simulink model "laser_cnc_camera_pid"  (R2024a)
settings: Solver=ode23t  StartTime=0.0  StopTime=0.6  RelTol=1e-3
libraries: slpidlib x1
settings Model: Creator=Sir Kiru  LastModifiedBy=Sir Kiru

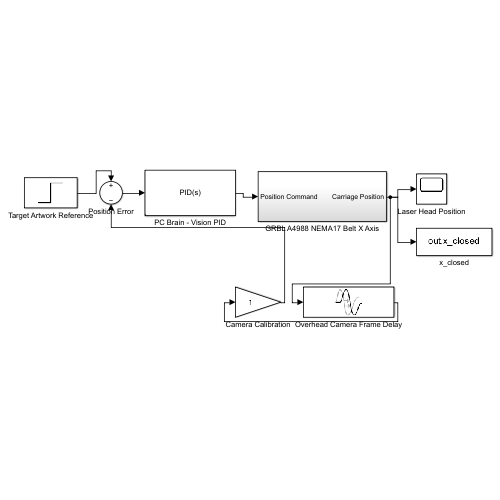
[thumbnail: Simulink's stored preview of the top-level diagram]
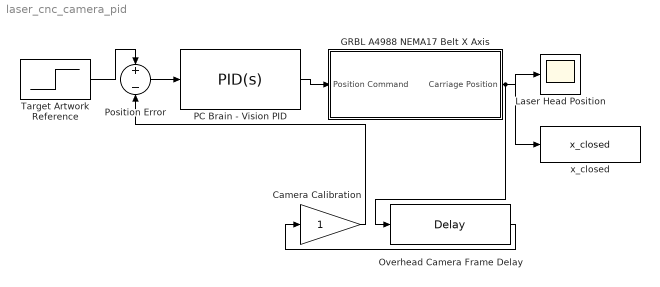
== system laser_cnc_camera_pid ==
  Camera Calibration : Gain
  GRBL A4988 NEMA17 Belt X Axis : Subsystem
  Laser Head Position : Scope
  Overhead Camera Frame Delay : TransportDelay  DelayTime=0.02
  PC Brain - Vision PID : slpidlib/PID Controller  Controller=PID  Form=Parallel  TimeDomain=Continuous-time  UseExternalTs=off  SampleTime=-1  IntegratorMethod=Forward Euler  FilterMethod=Forward Euler  ControllerParametersSource=internal  P=9  I=6  UseKiTs=off  D=0.16  UseExternalDerivativeSource=off  N=100  UseFilter=on  TunerSelectOption=Transfer Function Based (PID Tuner App)  InitialConditionSource=internal  InitialConditionForIntegrator=0  InitialConditionForFilter=0  DifferentiatorICPrevScaledInput=0  ExternalReset=none  TrackingMode=off  Kt=1  LimitOutput=off  SatLimitsSource=internal  UpperSaturationLimit=inf  LowerSaturationLimit=-inf  LinearizeAsGain=on  AntiWindupMode=none  Kb=1  LimitIntegrator=off  UpperIntegratorSaturationLimit=inf  LowerIntegratorSaturationLimit=-inf  POutMin=[]  POutMax=[]  IOutMin=[]  IOutMax=[]  DOutMin=[]  DOutMax=[]  NOutMin=[]  NOutMax=[]  SumOutMin=[]  SumOutMax=[]  SaturationOutMin=[]  SaturationOutMax=[]  PParamMin=[]  PParamMax=[]  IParamMin=[]  IParamMax=[]  DParamMin=[]  DParamMax=[]  NParamMin=[]  NParamMax=[]  KbParamMin=[]  KbParamMax=[]  KtParamMin=[]  KtParamMax=[]  KbOutMin=[]  KbOutMax=[]  KtOutMin=[]  KtOutMax=[]  IntegratorOutMin=[]  IntegratorOutMax=[]  FilterOutMin=[]  FilterOutMax=[]  SumI1OutMin=[]  SumI1OutMax=[]  SumI2OutMin=[]  SumI2OutMax=[]  SumI3OutMin=[]  SumI3OutMax=[]  SumI4OutMin=[]  SumI4OutMax=[]  SumDOutMin=[]  SumDOutMax=[]  DifferentiatorOutMin=[]  DifferentiatorOutMax=[]  FilterDiffOutCoefMin=[]  FilterDiffOutCoefMax=[]  ReciprocalOutMin=[]  ReciprocalOutMax=[]  SumDenOutMin=[]  SumDenOutMax=[]  SumNumOutMin=[]  SumNumOutMax=[]  DivideOutMin=[]  DivideOutMax=[]  UdiffTsProdOutMin=[]  UdiffTsProdOutMax=[]  NTsProdOutMin=[]  NTsProdOutMax=[]  UintegralTsProdOutMin=[]  UintegralTsProdOutMax=[]  UngainTsProdOutMin=[]  UngainTsProdOutMax=[]  ClampingZeroOutDataTypeStr=Inherit: Inherit via back propagation  ClampingZeroOutMin=[]  ClampingZeroOutMax=[]  FilterDenConstantOutDataTypeStr=Inherit: Inherit via back propagation  FilterDenConstantOutMin=[]  FilterDenConstantOutMax=[]  PCopyOutDataTypeStr=Inherit: Inherit via back propagation  PCopyOutMin=[]  PCopyOutMax=[]  NCopyOutDataTypeStr=Inherit: Inherit via back propagation  NCopyOutMin=[]  NCopyOutMax=[]  IntegratorContinuousStateAttributes=''  IntegratorStateMustResolveToSignalObject=off  IntegratorRTWStateStorageClass=Auto  FilterContinuousStateAttributes=''  FilterStateMustResolveToSignalObject=off  FilterRTWStateStorageClass=Auto  ParallelPVariant=InternalParameters  IdealPVariant=Disabled  IVariant=InternalParameters  DVariant=InternalParameters  IntegratorVariant=Continuous  SatVariant=Disabled  AWVariant=Passthrough  PCopyVariant=Disabled  TRVariant=Disabled  FdbkBlocksVariant=Forward  IdealPFdbkVariant=Disabled  SatFdbkVariant=Disabled  DerivativeFilterVariant=ContFilter  NVariant=InternalParameters  NCopyVariant=Disabled  FilterICVariant=InternalICsFilter  IntegratorICVariant=InternalICs  ExternalResetVariant=Disabled  TRSumVariant=Passthrough  SumFdbkVariant=Disabled  SumVariant=Sum_PID  TsampFilterVariant=InternalTs  TsampNgainVariant=Passthrough  TsampIntegralVariant=Disabled_SignalSpec  ExternalSaturationOutDataTypeStr=Inherit: Same as second input  DerivativeSourceVariant=ErrorSignal
  Position Error : Sum  Inputs=+-
  Target Artwork Reference : Step  Time=0.05  After=0.05  SampleTime=0
  x_closed : ToWorkspace  VariableName=x_closed  SaveFormat=Structure With Time  SampleTime=-1
  wires:
  Target Artwork Reference/1 -> Position Error/1
  Position Error/1 -> PC Brain - Vision PID/1
  PC Brain - Vision PID/1 -> GRBL A4988 NEMA17 Belt X Axis/1(Position Command)
  GRBL A4988 NEMA17 Belt X Axis/1(Carriage Position) -> Laser Head Position/1, x_closed/1, Overhead Camera Frame Delay/1
  Overhead Camera Frame Delay/1 -> Camera Calibration/1
  Camera Calibration/1 -> Position Error/2

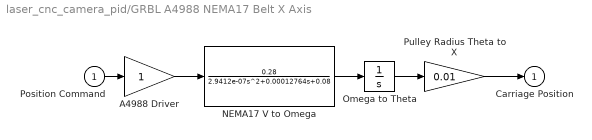
== system laser_cnc_camera_pid/GRBL A4988 NEMA17 Belt X Axis ==
  Position Command : Inport
  A4988 Driver : Gain
  NEMA17 V to Omega : TransferFcn  Numerator=[0.28]  Denominator=[2.9412e-07 0.00012764 0.08]
  Omega to Theta : Integrator
  Pulley Radius Theta to X : Gain  Gain=0.01
  Carriage Position : Outport
  wires:
  Position Command/1 -> A4988 Driver/1
  A4988 Driver/1 -> NEMA17 V to Omega/1
  NEMA17 V to Omega/1 -> Omega to Theta/1
  Omega to Theta/1 -> Pulley Radius Theta to X/1
  Pulley Radius Theta to X/1 -> Carriage Position/1
